simulink model "SimpleAcquisition_16ch_2014a_MI_errP"  (R2014a)
settings: Solver=FixedStepDiscrete  StartTime=0.0  StopTime=inf  FixedStep=1/512  RelTol=1e-3
undefined symbols (not defined in the file or in its folder): currentCFG_SimpleAcquisition_16ch_2014a_MI_errP_UB, UB
libraries: dspsigattribs x1, Tools x1, gtecHighspeedLib x1, gUSBamplib x1
settings Model: Creator=Leonardo  LastModifiedBy=Leonardo
settings DebuggingCC: MergeDetectMultiDrivingBlocksExec=error  FrameProcessingCompatibilityMsg=error

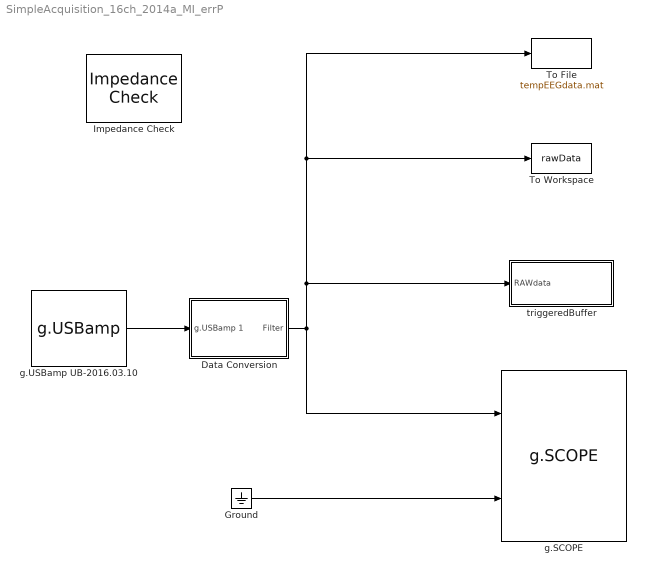
== system SimpleAcquisition_16ch_2014a_MI_errP ==
  "Data Conversion " : Subsystem
  Ground : Ground
  Impedance Check : Tools/Impedance Check
  To File : ToFile  Filename=tempEEGdata.mat  SaveFormat=Timeseries
  To Workspace : ToWorkspace  VariableName=rawData  SaveFormat=Timeseries  SampleTime=-1
  g.SCOPE : gtecHighspeedLib/g.SCOPE
  g.USBamp UB-2016.03.10 : gUSBamplib/g.USBamp  Priority=1  cfg=currentCFG_SimpleAcquisition_16ch_2014a_MI_errP_UB-2016.03.10.cfg  snr=UB-2016.03.10
  triggeredBuffer : Subsystem
      mask help:
      | Applies freq filters (1-10 Hz passband) and 1s buffering.
      | Each time it is triggered, buffered data is returned to workspace.
      mask init:
      | fs=512;
      | MIbufferLength=.4;
      | errPbufferLength=5;
  wires:
  Ground/1 -> g.SCOPE/2
  "Data Conversion "/1(Filter) -> triggeredBuffer/1(RAWdata), To File/1, To Workspace/1, g.SCOPE/1
  g.USBamp UB-2016.03.10/1 -> "Data Conversion "/1(g.USBamp 1)

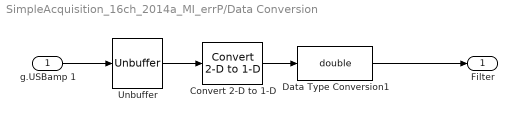
== system SimpleAcquisition_16ch_2014a_MI_errP/Data Conversion  ==
  g.USBamp 1 : Inport  Priority=2
  Convert 2-D to 1-D : dspsigattribs/Convert 2-D to 1-D
  Data Type Conversion1 : DataTypeConversion  OutDataTypeStr=double
  Unbuffer : Unbuffer  SampleBasedProcessing=Same as frame based
  Filter : Outport
  wires:
  g.USBamp 1/1 -> Unbuffer/1
  Unbuffer/1 -> Convert 2-D to 1-D/1
  Convert 2-D to 1-D/1 -> Data Type Conversion1/1
  Data Type Conversion1/1 -> Filter/1

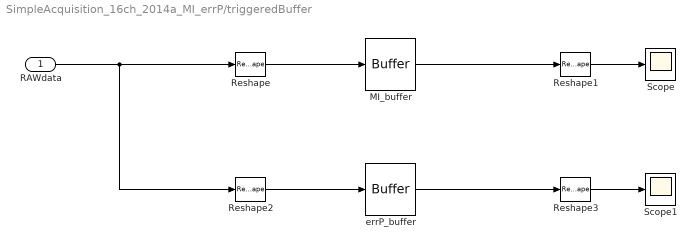
== system SimpleAcquisition_16ch_2014a_MI_errP/triggeredBuffer ==
  RAWdata : Inport
  MI_buffer : Buffer  N=round(fs*MIbufferLength)  V=round(fs*MIbufferLength)-1  TreatMby1Signals=One channel
  Reshape : Reshape  OutputDimensionality=Row vector (2-D)
  Reshape1 : Reshape
  Reshape2 : Reshape  OutputDimensionality=Row vector (2-D)
  Reshape3 : Reshape
  Scope : Scope
  Scope1 : Scope
  errP_buffer : Buffer  N=round(fs*errPbufferLength)  V=round(fs*errPbufferLength)-1  TreatMby1Signals=One channel
  wires:
  MI_buffer/1 -> Reshape1/1
  Reshape1/1 -> Scope/1
  Reshape/1 -> MI_buffer/1
  RAWdata/1 -> Reshape2/1, Reshape/1
  errP_buffer/1 -> Reshape3/1
  Reshape3/1 -> Scope1/1
  Reshape2/1 -> errP_buffer/1
